simulink model "Sim_4Bus_Chain_0d5_SG"  (R2020b)
settings: Solver=FixedStepAuto  StartTime=0  StopTime=10  FixedStep=Ts  RelTol=1e-3
values from neighbouring files (symbols this model uses):
  OtherInputs =     [matlab.mat]
  Ts = 1/Fs    [Main.m]    (also in main.m; matlab.mat = 3.33333333333e-05)
  Wbase = data.basic.Fbase*2*pi    [ConvertExcelFiles.m]    (also in Main.m = Fbase*2*pi; convertExcelFiles.m; main.m = W0; matlab.mat = 376.991118431)
  x_e =     [matlab.mat]
  Ybase = 1/Zbase    [Main.m]    (also in matlab.mat = 1000000000)
  Zbase = Sbase/Ibase    [Main.m]    (also in matlab.mat = 1e-09)
undefined symbols (not defined in the file or in its folder): DeviceDiscreDamping, DevicePara, DevicePowerFlow, DeviceType
libraries: powerlib x20, SimplexPS x12
settings Model: Creator=admin_user  LastModifiedBy=admin_user

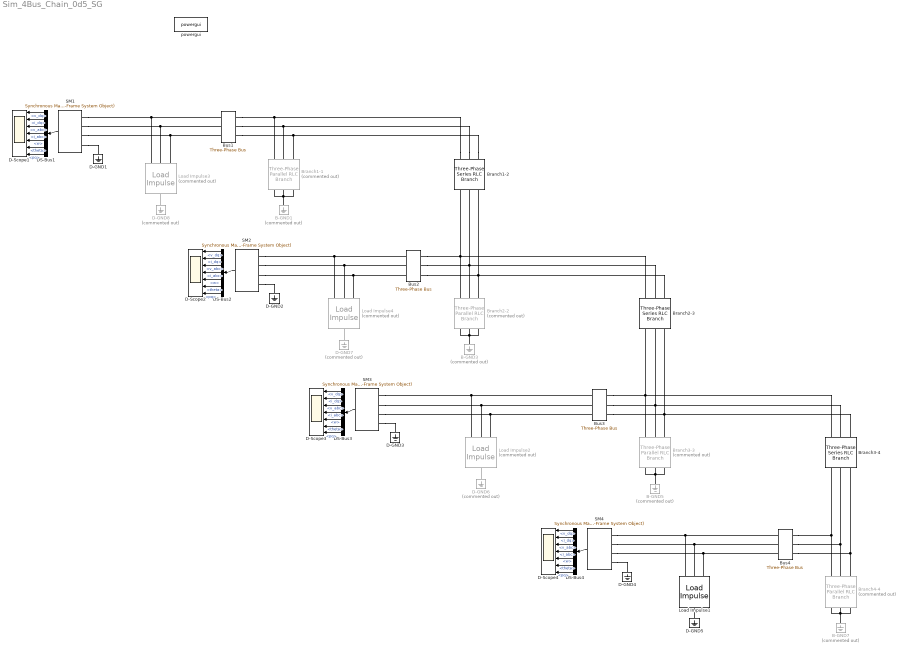
== system Sim_4Bus_Chain_0d5_SG ==
  B-GND{1,3,5,7} (4 alike) : powerlib/Elements/Ground  Commented=on  LConnTagsString=a
  Branch1-1 : powerlib/Elements/Three-Phase Parallel RLC Branch  Commented=on  LConnTagsString=A|B|C  RConnTagsString=A|B|C  BranchType=C  Resistance=(Inf)*Zbase  Inductance=1e-3  Capacitance=(0.001)*Ybase/Wbase  Measurements=None
      settings: SourceProductBaseCode=PS
  Branch1-2 : powerlib/Elements/Three-Phase Series RLC Branch  LConnTagsString=A|B|C  RConnTagsString=A|B|C  BranchType=RL  Resistance=(0.05)*Zbase  Inductance=(0.5)*Zbase/Wbase  Capacitance=1e-6  Measurements=None
  Branch2-2 : powerlib/Elements/Three-Phase Parallel RLC Branch  Commented=on  LConnTagsString=A|B|C  RConnTagsString=A|B|C  BranchType=C  Resistance=(Inf)*Zbase  Inductance=1e-3  Capacitance=(0.001)*Ybase/Wbase  Measurements=None
      settings: SourceProductBaseCode=PS
  Branch2-3 : powerlib/Elements/Three-Phase Series RLC Branch  LConnTagsString=A|B|C  RConnTagsString=A|B|C  BranchType=RL  Resistance=(0.05)*Zbase  Inductance=(0.5)*Zbase/Wbase  Capacitance=1e-6  Measurements=None
  Branch3-3 : powerlib/Elements/Three-Phase Parallel RLC Branch  Commented=on  LConnTagsString=A|B|C  RConnTagsString=A|B|C  BranchType=C  Resistance=(Inf)*Zbase  Inductance=1e-3  Capacitance=(0.001)*Ybase/Wbase  Measurements=None
      settings: SourceProductBaseCode=PS
  Branch3-4 : powerlib/Elements/Three-Phase Series RLC Branch  LConnTagsString=A|B|C  RConnTagsString=A|B|C  BranchType=RL  Resistance=(0.05)*Zbase  Inductance=(0.5)*Zbase/Wbase  Capacitance=1e-6  Measurements=None
  Branch4-4 : powerlib/Elements/Three-Phase Parallel RLC Branch  Commented=on  LConnTagsString=A|B|C  RConnTagsString=A|B|C  BranchType=C  Resistance=(Inf)*Zbase  Inductance=1e-3  Capacitance=(0.001)*Ybase/Wbase  Measurements=None
      settings: SourceProductBaseCode=PS
  Bus{1..4} (4 alike) : SimplexPS/Three-Phase Bus  Vbase=1  Sbase=1
  D-GND{1..5} (5 alike) : powerlib/Elements/Ground  LConnTagsString=a
  D-GND6 : powerlib/Elements/Ground  Commented=on  LConnTagsString=a
  D-GND7 : powerlib/Elements/Ground  Commented=on  LConnTagsString=a
  D-GND8 : powerlib/Elements/Ground  Commented=on  LConnTagsString=a
  D-Scope{1..4} (4 alike) : Scope  NumInputPorts=7
  DS-Bus{1..4} (4 alike) : BusSelector  OutputSignals=v_dq,i_dq,v_abc,i_abc,w,theta,pq
  Load Impulse1 : SimplexPS/Load Impulse  t0=5  dt=1/60*4  R=1e-9*Zbase
  Load Impulse2 : SimplexPS/Load Impulse  Commented=on  t0=5  dt=1/60*4  R=1e-9*Zbase
  Load Impulse3 : SimplexPS/Load Impulse  Commented=on  t0=5  dt=1/60*4  R=1e-9*Zbase
  Load Impulse4 : SimplexPS/Load Impulse  Commented=on  t0=5  dt=1/60*4  R=1e-9*Zbase
  SM1 : SimplexPS/Synchronous Machine (dq-Frame System Object)  Ts=Ts  Sbase=Sbase  Vbase=Vbase  Wbase=Wbase  DeviceType=DeviceType{1}  DevicePara=DevicePara{1}  PowerFlow=DevicePowerFlow{1}  x0=x_e{1}  OtherInputs=OtherInputs{1}  DiscreMethod=Hybrid Trapezoidal  EnableInsideModification=off  DiscreDampingFlag=on  DiscreDampingValue=DeviceDiscreDamping{1}  LinearizationTimes=1  DirectFeedthrough=off
  SM2 : SimplexPS/Synchronous Machine (dq-Frame System Object)  Ts=Ts  Sbase=Sbase  Vbase=Vbase  Wbase=Wbase  DeviceType=DeviceType{2}  DevicePara=DevicePara{2}  PowerFlow=DevicePowerFlow{2}  x0=x_e{2}  OtherInputs=OtherInputs{2}  DiscreMethod=Hybrid Trapezoidal  EnableInsideModification=off  DiscreDampingFlag=on  DiscreDampingValue=DeviceDiscreDamping{2}  LinearizationTimes=1  DirectFeedthrough=off
  SM3 : SimplexPS/Synchronous Machine (dq-Frame System Object)  Ts=Ts  Sbase=Sbase  Vbase=Vbase  Wbase=Wbase  DeviceType=DeviceType{3}  DevicePara=DevicePara{3}  PowerFlow=DevicePowerFlow{3}  x0=x_e{3}  OtherInputs=OtherInputs{3}  DiscreMethod=Hybrid Trapezoidal  EnableInsideModification=off  DiscreDampingFlag=on  DiscreDampingValue=DeviceDiscreDamping{3}  LinearizationTimes=1  DirectFeedthrough=off
  SM4 : SimplexPS/Synchronous Machine (dq-Frame System Object)  Ts=Ts  Sbase=Sbase  Vbase=Vbase  Wbase=Wbase  DeviceType=DeviceType{4}  DevicePara=DevicePara{4}  PowerFlow=DevicePowerFlow{4}  x0=x_e{4}  OtherInputs=OtherInputs{4}  DiscreMethod=Hybrid Trapezoidal  EnableInsideModification=off  DiscreDampingFlag=on  DiscreDampingValue=DeviceDiscreDamping{4}  LinearizationTimes=1  DirectFeedthrough=off
  powergui : powerlib/powergui  Priority=1  SimulationMode=Discrete  SampleTime=Ts  frequency=60  Iterations=50  frequencyindice=0  Pbase=100e6  ErrMax=1e-4  UnitsV=kV  UnitsW=MW  buscounter=0  FunctionMessages=off  echomessages=off  EnableUseOfTLC=off  CurrentSourceSwitches=off  DisableSnubberDevices=off  DisableRonSwitches=off  DisableVfSwitches=off  DisplayEquations=off  AutomaticDiscreteSolvers=off  SolverType=Tustin/Backward Euler (TBE)  Interpol=off  ExternalGateDelay=off  methode=off  Ts=100  x0status=blocks  SPID=on  SwTol=0  HookPort=off  NonlinearTolerance=1e-4  nMaxIteration=100  ContinueOnMaxIteration=off  RestoreLinks=warning  ResistiveCurrentMeasurement=off  Frange=[0:2:500]  Ylog=off  Xlog=on  ShowGrid=off  save=off  variable=ZData  structure=0  ZoomFFT=off  StartTime=0.0  cycles=1  DisplayStyle=1  fundamental=60  FreqAxis=off  MaxFrequency=1000  frequencyindicesteady=1  RmsSteady=1  display=off
  wires:
  SM1/1 -> DS-Bus1/1
  DS-Bus1/1 -> D-Scope1/1  "<v_dq>"
  DS-Bus1/2 -> D-Scope1/2  "<i_dq>"
  DS-Bus1/3 -> D-Scope1/3  "<v_abc>"
  DS-Bus1/4 -> D-Scope1/4  "<i_abc>"
  DS-Bus1/5 -> D-Scope1/5  "<w>"
  DS-Bus1/6 -> D-Scope1/6  "<theta>"
  DS-Bus1/7 -> D-Scope1/7  "<pq>"
  SM2/1 -> DS-Bus2/1
  DS-Bus2/1 -> D-Scope2/1  "<v_dq>"
  DS-Bus2/2 -> D-Scope2/2  "<i_dq>"
  DS-Bus2/3 -> D-Scope2/3  "<v_abc>"
  DS-Bus2/4 -> D-Scope2/4  "<i_abc>"
  DS-Bus2/5 -> D-Scope2/5  "<w>"
  DS-Bus2/6 -> D-Scope2/6  "<theta>"
  DS-Bus2/7 -> D-Scope2/7  "<pq>"
  SM3/1 -> DS-Bus3/1
  DS-Bus3/1 -> D-Scope3/1  "<v_dq>"
  DS-Bus3/2 -> D-Scope3/2  "<i_dq>"
  DS-Bus3/3 -> D-Scope3/3  "<v_abc>"
  DS-Bus3/4 -> D-Scope3/4  "<i_abc>"
  DS-Bus3/5 -> D-Scope3/5  "<w>"
  DS-Bus3/6 -> D-Scope3/6  "<theta>"
  DS-Bus3/7 -> D-Scope3/7  "<pq>"
  SM4/1 -> DS-Bus4/1
  DS-Bus4/1 -> D-Scope4/1  "<v_dq>"
  DS-Bus4/2 -> D-Scope4/2  "<i_dq>"
  DS-Bus4/3 -> D-Scope4/3  "<v_abc>"
  DS-Bus4/4 -> D-Scope4/4  "<i_abc>"
  DS-Bus4/5 -> D-Scope4/5  "<w>"
  DS-Bus4/6 -> D-Scope4/6  "<theta>"
  DS-Bus4/7 -> D-Scope4/7  "<pq>"
  connections:
  SM1/LConn4 -- D-GND1/LConn1
  SM2/LConn4 -- D-GND2/LConn1
  SM3/LConn4 -- D-GND3/LConn1
  SM4/LConn4 -- D-GND4/LConn1
  Branch1-1/RConn1 -- Branch1-1/RConn2 -- Branch1-1/RConn3 -- B-GND1/LConn1
  Branch2-2/RConn1 -- Branch2-2/RConn2 -- Branch2-2/RConn3 -- B-GND3/LConn1
  Branch3-3/RConn1 -- Branch3-3/RConn2 -- Branch3-3/RConn3 -- B-GND5/LConn1
  Branch4-4/RConn1 -- Branch4-4/RConn2 -- Branch4-4/RConn3 -- B-GND7/LConn1
  Branch1-2/RConn1 -- Bus2/RConn1 -- Branch2-2/LConn1 -- Branch2-3/LConn1
  Branch1-2/RConn2 -- Bus2/RConn2 -- Branch2-2/LConn2 -- Branch2-3/LConn2
  Branch1-2/RConn3 -- Bus2/RConn3 -- Branch2-2/LConn3 -- Branch2-3/LConn3
  Branch1-2/LConn1 -- Bus1/RConn1 -- Branch1-1/LConn1
  Branch1-2/LConn2 -- Bus1/RConn2 -- Branch1-1/LConn2
  Branch1-2/LConn3 -- Bus1/RConn3 -- Branch1-1/LConn3
  Branch2-3/RConn1 -- Bus3/RConn1 -- Branch3-3/LConn1 -- Branch3-4/LConn1
  Branch2-3/RConn2 -- Bus3/RConn2 -- Branch3-3/LConn2 -- Branch3-4/LConn2
  Branch2-3/RConn3 -- Bus3/RConn3 -- Branch3-3/LConn3 -- Branch3-4/LConn3
  Branch3-4/RConn1 -- Bus4/RConn1 -- Branch4-4/LConn1
  Branch3-4/RConn2 -- Bus4/RConn2 -- Branch4-4/LConn2
  Branch3-4/RConn3 -- Bus4/RConn3 -- Branch4-4/LConn3
  SM1/LConn1 -- Load Impulse3/LConn1 -- Bus1/LConn1
  SM1/LConn2 -- Load Impulse3/LConn2 -- Bus1/LConn2
  SM1/LConn3 -- Load Impulse3/LConn3 -- Bus1/LConn3
  SM2/LConn1 -- Load Impulse4/LConn1 -- Bus2/LConn1
  SM2/LConn2 -- Load Impulse4/LConn2 -- Bus2/LConn2
  SM2/LConn3 -- Load Impulse4/LConn3 -- Bus2/LConn3
  SM3/LConn1 -- Load Impulse2/LConn1 -- Bus3/LConn1
  SM3/LConn2 -- Load Impulse2/LConn2 -- Bus3/LConn2
  SM3/LConn3 -- Load Impulse2/LConn3 -- Bus3/LConn3
  SM4/LConn1 -- Load Impulse1/LConn1 -- Bus4/LConn1
  SM4/LConn2 -- Load Impulse1/LConn2 -- Bus4/LConn2
  SM4/LConn3 -- Bus4/LConn3 -- Load Impulse1/LConn3
  D-GND8/LConn1 -- Load Impulse3/RConn1
  D-GND5/LConn1 -- Load Impulse1/RConn1
  D-GND6/LConn1 -- Load Impulse2/RConn1
  D-GND7/LConn1 -- Load Impulse4/RConn1
